simulink model "SCC_my"  (R2013a)
settings: Solver=ode45  StartTime=0.0  StopTime=10.0  RelTol=1e-3
libraries: simulink x2
settings Model: Creator=IVDL  LastModifiedBy=IVDL

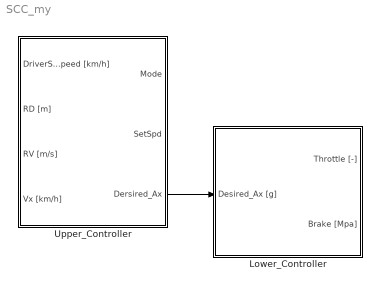
== system SCC_my ==
  Lower_Controller : Subsystem
  Upper_Controller : Subsystem
  wires:
  Upper_Controller/3(Dersired_Ax) -> Lower_Controller/1(Desired_Ax [g])

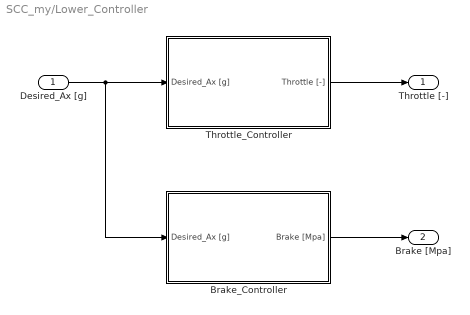
== system SCC_my/Lower_Controller ==
  Desired_Ax [g] : Inport
  Brake_Controller : Subsystem
  Throttle_Controller : Subsystem
  Throttle [-] : Outport
  Brake [Mpa] : Outport  Port=2
  wires:
  Desired_Ax [g]/1 -> Brake_Controller/1(Desired_Ax [g]), Throttle_Controller/1(Desired_Ax [g])
  Throttle_Controller/1(Throttle [-]) -> Throttle [-]/1
  Brake_Controller/1(Brake [Mpa]) -> Brake [Mpa]/1

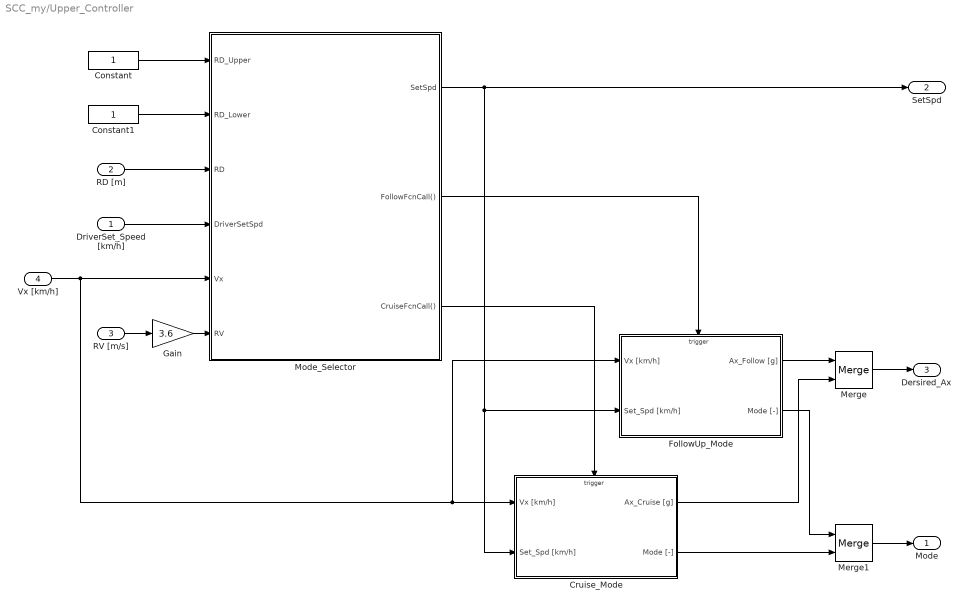
== system SCC_my/Upper_Controller ==
  DriverSet_Speed [km/h] : Inport
  RD [m] : Inport  Port=2
  RV [m/s] : Inport  Port=3
  Vx [km/h] : Inport  Port=4
  Constant : Constant
  Constant1 : Constant
  Cruise_Mode : Subsystem  TreatAsAtomicUnit=on
  FollowUp_Mode : Subsystem  TreatAsAtomicUnit=on
  Gain : Gain  Gain=3.6
  Merge : Merge
  Merge1 : Merge
  Mode_Selector : Stateflow chart  TreatAsAtomicUnit=on
  Mode : Outport
  SetSpd : Outport  Port=2
  Dersired_Ax : Outport  Port=3
  wires:
  Constant/1 -> Mode_Selector/1(RD_Upper)
  Constant1/1 -> Mode_Selector/2(RD_Lower)
  Vx [km/h]/1 -> Cruise_Mode/1(Vx [km/h]), FollowUp_Mode/1(Vx [km/h]), Mode_Selector/5(Vx)
  RV [m/s]/1 -> Gain/1
  DriverSet_Speed [km/h]/1 -> Mode_Selector/4(DriverSetSpd)
  RD [m]/1 -> Mode_Selector/3(RD)
  Gain/1 -> Mode_Selector/6(RV)
  Mode_Selector/2(FollowFcnCall()) -> FollowUp_Mode/Trigger
  Mode_Selector/3(CruiseFcnCall()) -> Cruise_Mode/Trigger
  Mode_Selector/1(SetSpd) -> FollowUp_Mode/2(Set_Spd [km/h]), Cruise_Mode/2(Set_Spd [km/h]), SetSpd/1
  Cruise_Mode/1(Ax_Cruise [g]) -> Merge/2
  Merge/1 -> Dersired_Ax/1
  Merge1/1 -> Mode/1
  FollowUp_Mode/2(Mode [-]) -> Merge1/1
  Cruise_Mode/2(Mode [-]) -> Merge1/2
  FollowUp_Mode/1(Ax_Follow [g]) -> Merge/1

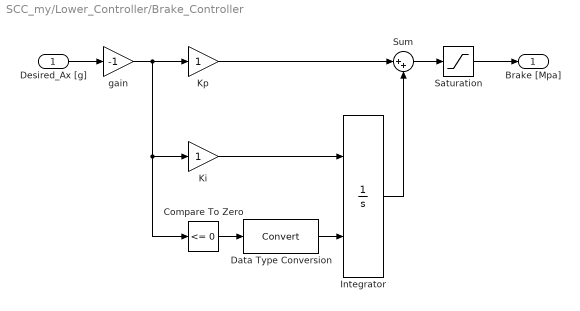
== system SCC_my/Lower_Controller/Brake_Controller ==
  Desired_Ax [g] : Inport
  Compare To Zero : simulink/Logic and Bit Operations/Compare To Zero  relop=<=  OutDataTypeStr=boolean
  Data Type Conversion : DataTypeConversion
  Integrator : Integrator  ExternalReset=rising
  Ki : Gain
  Kp : Gain
  Saturation : Saturate  LowerLimit=0
  Sum : Sum  Inputs=|++
  gain : Gain  Gain=-1
  Brake [Mpa] : Outport
  wires:
  Desired_Ax [g]/1 -> gain/1
  Compare To Zero/1 -> Data Type Conversion/1
  Data Type Conversion/1 -> Integrator/2
  Ki/1 -> Integrator/1
  Integrator/1 -> Sum/2
  Kp/1 -> Sum/1
  Sum/1 -> Saturation/1
  Saturation/1 -> Brake [Mpa]/1
  gain/1 -> Ki/1, Compare To Zero/1, Kp/1

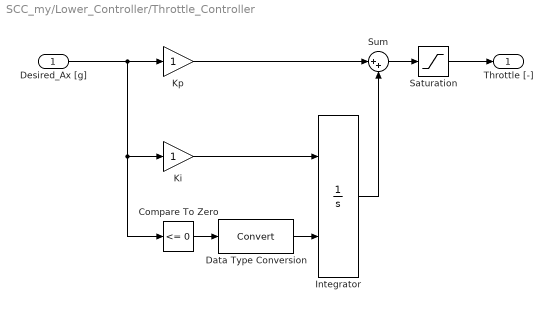
== system SCC_my/Lower_Controller/Throttle_Controller ==
  Desired_Ax [g] : Inport
  Compare To Zero : simulink/Logic and Bit Operations/Compare To Zero  relop=<=  OutDataTypeStr=boolean
  Data Type Conversion : DataTypeConversion
  Integrator : Integrator  ExternalReset=rising
  Ki : Gain
  Kp : Gain
  Saturation : Saturate  UpperLimit=1  LowerLimit=0
  Sum : Sum  Inputs=|++
  Throttle [-] : Outport
  wires:
  Desired_Ax [g]/1 -> Ki/1, Compare To Zero/1, Kp/1
  Compare To Zero/1 -> Data Type Conversion/1
  Data Type Conversion/1 -> Integrator/2
  Ki/1 -> Integrator/1
  Integrator/1 -> Sum/2
  Kp/1 -> Sum/1
  Sum/1 -> Saturation/1
  Saturation/1 -> Throttle [-]/1

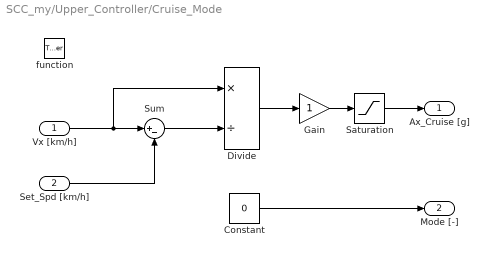
== system SCC_my/Upper_Controller/Cruise_Mode ==
  Vx [km/h] : Inport
  Set_Spd [km/h] : Inport  Port=2
  function : TriggerPort  TriggerType=function-call
  Constant : Constant  Value=0
  Divide : Product  Inputs=*/
  Gain : Gain
  Saturation : Saturate  UpperLimit=0.3  LowerLimit=-0.3
  Sum : Sum  Inputs=|+-
  Ax_Cruise [g] : Outport
  Mode [-] : Outport  Port=2
  wires:
  Vx [km/h]/1 -> Divide/1, Sum/1
  Set_Spd [km/h]/1 -> Sum/2
  Sum/1 -> Divide/2
  Divide/1 -> Gain/1
  Gain/1 -> Saturation/1
  Saturation/1 -> Ax_Cruise [g]/1
  Constant/1 -> Mode [-]/1

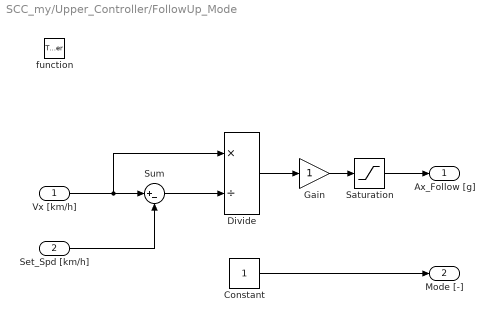
== system SCC_my/Upper_Controller/FollowUp_Mode ==
  Vx [km/h] : Inport
  Set_Spd [km/h] : Inport  Port=2
  function : TriggerPort  TriggerType=function-call
  Constant : Constant
  Divide : Product  Inputs=*/
  Gain : Gain
  Saturation : Saturate  UpperLimit=0.4  LowerLimit=-0.4
  Sum : Sum  Inputs=|+-
  Ax_Follow [g] : Outport
  Mode [-] : Outport  Port=2
  wires:
  Vx [km/h]/1 -> Divide/1, Sum/1
  Set_Spd [km/h]/1 -> Sum/2
  Sum/1 -> Divide/2
  Divide/1 -> Gain/1
  Gain/1 -> Saturation/1
  Constant/1 -> Mode [-]/1
  Saturation/1 -> Ax_Follow [g]/1

== stateflow chart SCC_my/Upper_Controller/Mode_Selector ==
  state Cruise_Mode
    du, en : TVSpd = RV+Vx;
    du : send(CruiseFcnCall);
    du : SetSpd = DriverSetSpd;
  state FollowUp_Mode
    du, en : TVSpd = RV+Vx;
    du : send(FollowFcnCall);
    du : SetSpd = TVSpd;
  (default) -> Cruise_Mode
  Cruise_Mode -> FollowUp_Mode : [ (RD<=RD_Lower) & (DriverSetSpd >= TVSpd) ]
  FollowUp_Mode -> Cruise_Mode : [ (RD>RD_Upper) | (DriverSetSpd< TVSpd) ]
  data: RD_Upper input double; RD_Lower input double; RD input double; DriverSetSpd input double; SetSpd output double; Vx input double; RV input double; TVSpd local double
  events: FollowFcnCall output FUNCTION_CALL_EVENT; CruiseFcnCall output FUNCTION_CALL_EVENT
